simulink model "timer_s"  (R2023a)
settings: Solver=FixedStepAuto  StartTime=0.0  StopTime=10.0  FixedStep=0.01  RelTol=1e-3
settings Model: Creator=23208  LastModifiedBy=wkmiao

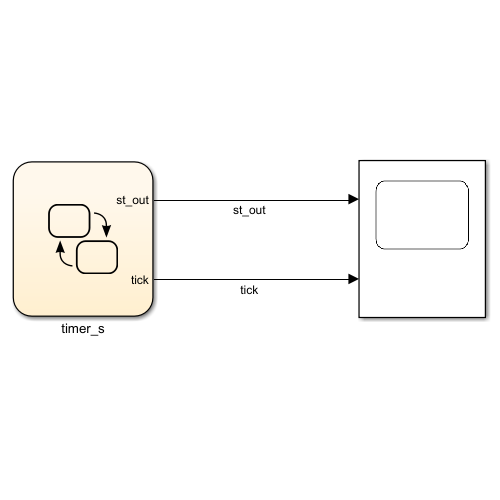
[thumbnail: Simulink's stored preview of the top-level diagram]
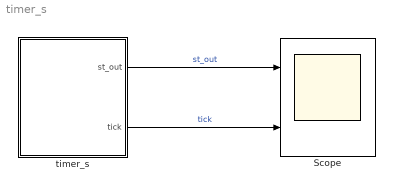
== system timer_s ==
  Scope : Scope  NumInputPorts=2
  timer_s : Stateflow chart  TreatAsAtomicUnit=on
  wires:
  timer_s/1(st_out) -> Scope/1  "st_out"
  timer_s/2(tick) -> Scope/2  "tick"

== stateflow chart timer_s/timer_s ==
  settings: updateMethod=CONTINUOUS  executeAtInitialization=1  initializeOutput=1
  state timer
    du:
    st_dot = 1;
    st_out = st;
  (default) -> timer : {
      | st=0
      | }
  timer -> timer : [st>=T]{tick=1;st=0;}
  data: st_out output double; st local; T local =2; tick output
  data st settings: updateMethod=SF_CONTINUOUS_TIME_DATA
